simulink subsystem "PID_gain_scheduling"  (R2024a)
settings: Solver=VariableStepAuto  StartTime=0.0  StopTime=10.0  RelTol=1e-3
undefined symbols (not defined in the file): K_PID_gain_scheduling, u_eq, z_stars
settings Model: Creator=Bocchio  LastModifiedBy=Bocchio

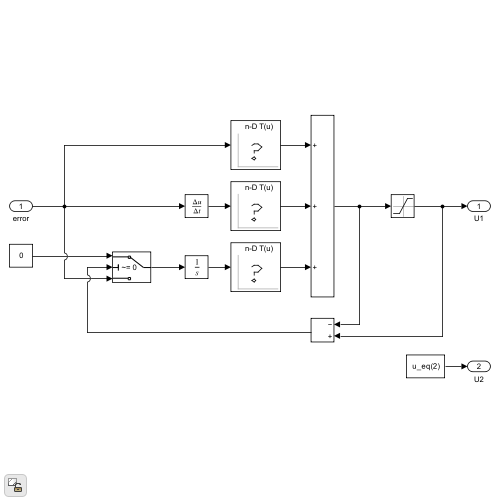
[thumbnail: Simulink's stored preview of the top-level diagram]
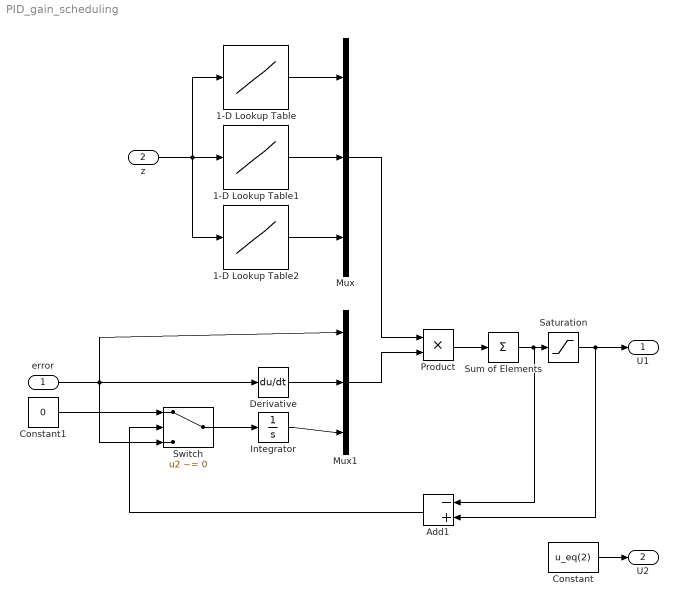
== system PID_gain_scheduling ==
  error : Inport
  z : Inport  Port=2
  1-D Lookup Table : Lookup_n-D  NumberOfTableDimensions=1  BreakpointsForDimension1=z_stars  Table=K_PID_gain_scheduling.Kp  InternalRulePriority=Speed  RndMeth=Simplest
  1-D Lookup Table1 : Lookup_n-D  NumberOfTableDimensions=1  BreakpointsForDimension1=z_stars  Table=K_PID_gain_scheduling.Kd  InternalRulePriority=Speed  RndMeth=Simplest
  1-D Lookup Table2 : Lookup_n-D  NumberOfTableDimensions=1  BreakpointsForDimension1=z_stars  Table=K_PID_gain_scheduling.Ki  InternalRulePriority=Speed  RndMeth=Simplest
  Add1 : Sum  Inputs=-+
  Constant : Constant  Value=u_eq(2)
  Constant1 : Constant  Value=0
  Derivative : Derivative  CoefficientInTFapproximation=1e6
  Integrator : Integrator
  Mux : Mux  Inputs=3
  Mux1 : Mux  Inputs=3
  Product : Product
  Saturation : Saturate  UpperLimit=1  LowerLimit=0
  Sum of Elements : Sum  Inputs=+
  Switch : Switch  Criteria=u2 ~= 0  SaturateOnIntegerOverflow=off  InputSameDT=off
  U1 : Outport
  U2 : Outport  Port=2
  wires:
  Constant/1 -> U2/1
  error/1 -> Derivative/1, Switch/3, Mux1/1
  Derivative/1 -> Mux1/2
  Sum of Elements/1 -> Add1/1, Saturation/1
  Switch/1 -> Integrator/1
  Add1/1 -> Switch/2
  Saturation/1 -> Add1/2, U1/1
  Constant1/1 -> Switch/1
  Integrator/1 -> Mux1/3
  z/1 -> 1-D Lookup Table2/1, 1-D Lookup Table1/1, 1-D Lookup Table/1
  1-D Lookup Table/1 -> Mux/1
  1-D Lookup Table1/1 -> Mux/2
  1-D Lookup Table2/1 -> Mux/3
  Mux/1 -> Product/1
  Product/1 -> Sum of Elements/1
  Mux1/1 -> Product/2
